simulink model "Uebung07_Aufgabe1_urspruengliche_Situation"  (R2017a)
settings: Solver=VariableStepAuto  StartTime=0.0  StopTime=10000  RelTol=1e-3  EnableMultiTasking=on
undefined symbols (not defined in the file or in its folder): calcElapsedTime, entity, m, n
settings Model: Creator=gome  LastModifiedBy=gome
settings OptimizationCC: LifeSpan=inf
settings DebuggingCC: SFUnexpectedBacktrackingDiag=warning  SFNoUnconditionalDefaultTransitionDiag=warning  SFExecutionAtInitializationDiag=none
settings GRTTargetCC: TargetLangStandard=C89/C90 (ANSI)  GeneratePreprocessorConditionals=Disable all
settings ConfigComp: CovMetricSettings=dw  CovHtmlReporting=on  CovSaveCumulativeToWorkspaceVar=on  CovSaveSingleToWorkspaceVar=on  CovExternalEMLEnable=off

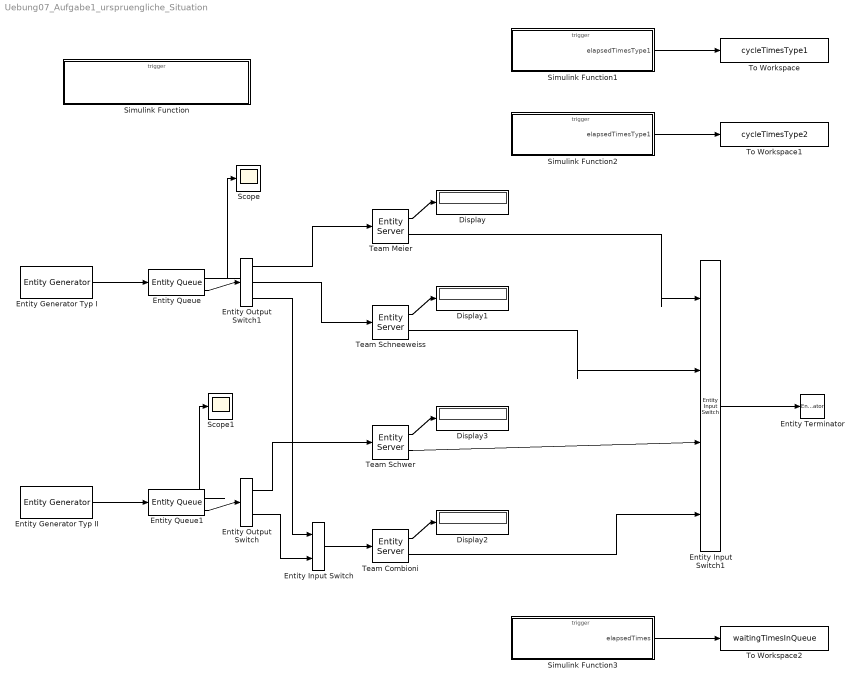
== system Uebung07_Aufgabe1_urspruengliche_Situation ==
  Display{,1..3} (4 alike) : Display
  Entity Input Switch : EntityInputSwitch  InputPortMessageModes=m,m  OutputPortMessageModes=m
  Entity Input Switch1 : EntityInputSwitch  InputPortMessageModes=m,m,m,m  OutputPortMessageModes=m  NumberInputPorts=4
      settings: InputPortMap=u1,u2,u3,u4
  Entity Output Switch : EntityOutputSwitch  InputPortMessageModes=m  OutputPortMessageModes=m,m  SwitchAttributeName=Attribute1
  Entity Output Switch1 : EntityOutputSwitch  InputPortMessageModes=m  OutputPortMessageModes=m,m,m  NumberOutputPorts=3  SwitchAttributeName=Attribute1
      settings: OutputPortMap=o0,o1,o2
  Entity Generator Typ I : EntityGenerator  OutputPortMessageModes=m  TimeSource=MATLAB action  IntergenerationTimeAction=dt = exprnd(0.333333);  GenerateAction=|  AttributeName=startTime|serviceTime|type  AttributeInitialValue=1|1|1  EntityType=Structured  EntityTypeName=Entity
      | entity.startTime = getCurrentSimTime;
      | entity.serviceTime = exprnd(0.25);
  Entity Generator Typ II : EntityGenerator  OutputPortMessageModes=m  TimeSource=MATLAB action  Period=36.3636  IntergenerationTimeAction=|  GenerateAction=|  AttributeName=startTime|serviceTime|type  AttributeInitialValue=1|1|2  EntityType=Structured  EntityTypeName=Entity
      IntergenerationTimeAction=|
      | persistent init
      | if isempty(init)
      |     init = 1;
      |     rng(845094850);
      | end
      | 
      | dt = exprnd(1.7143);
      GenerateAction=|
      | entity.startTime = getCurrentSimTime;
      | entity.serviceTime = exprnd(1);
  Entity Queue : EntityQueue  InputPortMessageModes=m  OutputPortMessageModes=n,m  Capacity=inf  ExitAction=calcElapsedTime(entity.startTime);  NumberEntitiesInBlock=on
      settings: OutputPortMap=o1,o5
  Entity Queue1 : EntityQueue  InputPortMessageModes=m  OutputPortMessageModes=n,m  Capacity=inf  ExitAction=calcElapsedTime(entity.startTime);  NumberEntitiesInBlock=on
      settings: OutputPortMap=o1,o5
  Entity Terminator : EntityTerminator  InputPortMessageModes=m  EntryAction=|
      | if entity.type == 1
      |     calcElapsedTime1(entity.startTime);
      | else
      |     calcElapsedTime2(entity.startTime);
      | end
  Scope : Scope
  Scope1 : Scope
  Simulink Function : Subsystem  TreatAsAtomicUnit=on
  Simulink Function1 : Subsystem  TreatAsAtomicUnit=on
  Simulink Function2 : Subsystem  TreatAsAtomicUnit=on
  Simulink Function3 : Subsystem  TreatAsAtomicUnit=on
  Team Combioni : EntityServer  InputPortMessageModes=m  OutputPortMessageModes=n,m  Capacity=1  ServiceTimeSource=Attribute  ServiceTimeAttributeName=serviceTime  Utilization=on
      settings: OutputPortMap=o5,o9
  Team Meier : EntityServer  InputPortMessageModes=m  OutputPortMessageModes=n,m  Capacity=1  ServiceTimeSource=Attribute  ServiceTimeAttributeName=serviceTime  Utilization=on
      settings: OutputPortMap=o5,o9
  Team Schneeweiss : EntityServer  InputPortMessageModes=m  OutputPortMessageModes=n,m  Capacity=1  ServiceTimeSource=Attribute  ServiceTimeAttributeName=serviceTime  Utilization=on
      settings: OutputPortMap=o5,o9
  Team Schwer : EntityServer  InputPortMessageModes=m  OutputPortMessageModes=n,m  Capacity=1  ServiceTimeSource=Attribute  ServiceTimeAttributeName=serviceTime  Utilization=on
      settings: OutputPortMap=o5,o9
  To Workspace : ToWorkspace  VariableName=cycleTimesType1  SaveFormat=Timeseries  SampleTime=-1
  To Workspace1 : ToWorkspace  VariableName=cycleTimesType2  SaveFormat=Timeseries  SampleTime=-1
  To Workspace2 : ToWorkspace  VariableName=waitingTimesInQueue  SaveFormat=Timeseries  SampleTime=-1
  wires:
  Entity Queue/2 -> Entity Output Switch1/1
  Entity Queue1/2 -> Entity Output Switch/1
  Entity Generator Typ II/1 -> Entity Queue1/1
  Entity Generator Typ I/1 -> Entity Queue/1
  Entity Output Switch1/1 -> Team Meier/1
  Entity Output Switch1/2 -> Team Schneeweiss/1
  Entity Input Switch/1 -> Team Combioni/1
  Entity Output Switch1/3 -> Entity Input Switch/1
  Entity Output Switch/2 -> Entity Input Switch/2
  Entity Output Switch/1 -> Team Schwer/1
  Team Meier/2 -> Entity Input Switch1/1
  Team Schneeweiss/2 -> Entity Input Switch1/2
  Team Schwer/2 -> Entity Input Switch1/3
  Team Combioni/2 -> Entity Input Switch1/4
  Entity Input Switch1/1 -> Entity Terminator/1
  Simulink Function1/1(elapsedTimesType1) -> To Workspace/1
  Team Meier/1 -> Display/1
  Team Combioni/1 -> Display2/1
  Team Schwer/1 -> Display3/1
  Team Schneeweiss/1 -> Display1/1
  Simulink Function2/1(elapsedTimesType1) -> To Workspace1/1
  Simulink Function3/1(elapsedTimes) -> To Workspace2/1
  Entity Queue/1 -> Scope/1
  Entity Queue1/1 -> Scope1/1

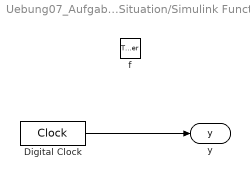
== system Uebung07_Aufgabe1_urspruengliche_Situation/Simulink Function ==
  f : TriggerPort  TriggerType=function-call  IsSimulinkFunction=on  FunctionName=getCurrentSimTime  VariantControl=Variant
  Digital Clock : DigitalClock  SampleTime=-1
  y : ArgOut  DisableCoverage=on  ArgumentName=y
  wires:
  Digital Clock/1 -> y/1

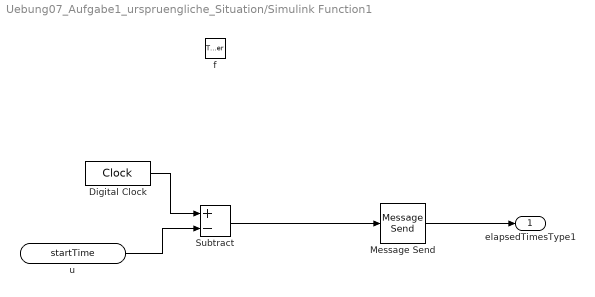
== system Uebung07_Aufgabe1_urspruengliche_Situation/Simulink Function1 ==
  f : TriggerPort  TriggerType=function-call  IsSimulinkFunction=on  FunctionName=calcElapsedTime1  VariantControl=Variant
  Digital Clock : DigitalClock  SampleTime=-1
  Message Send : MessageSend  OutputPortMessageModes=m
      settings: InputPortMap=u1
  Subtract : Sum  Inputs=+-
  u : ArgIn  DisableCoverage=on  ArgumentName=startTime
  elapsedTimesType1 : Outport
  wires:
  Message Send/1 -> elapsedTimesType1/1
  Subtract/1 -> Message Send/1
  Digital Clock/1 -> Subtract/1
  u/1 -> Subtract/2

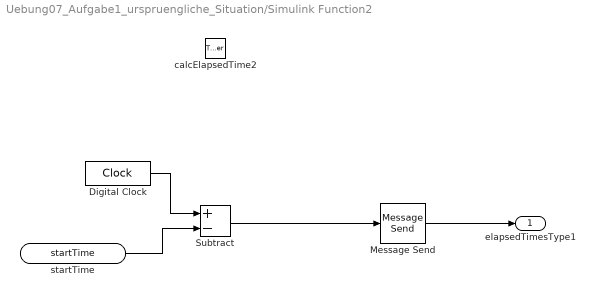
== system Uebung07_Aufgabe1_urspruengliche_Situation/Simulink Function2 ==
  calcElapsedTime2 : TriggerPort  TriggerType=function-call  IsSimulinkFunction=on  FunctionName=calcElapsedTime2  VariantControl=Variant
  Digital Clock : DigitalClock  SampleTime=-1
  Message Send : MessageSend  OutputPortMessageModes=m
      settings: InputPortMap=u1
  Subtract : Sum  Inputs=+-
  startTime : ArgIn  DisableCoverage=on  ArgumentName=startTime
  elapsedTimesType1 : Outport
  wires:
  Message Send/1 -> elapsedTimesType1/1
  Subtract/1 -> Message Send/1
  Digital Clock/1 -> Subtract/1
  startTime/1 -> Subtract/2

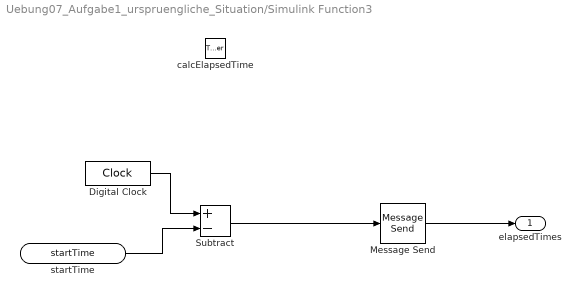
== system Uebung07_Aufgabe1_urspruengliche_Situation/Simulink Function3 ==
  calcElapsedTime : TriggerPort  TriggerType=function-call  IsSimulinkFunction=on  FunctionName=calcElapsedTime  VariantControl=Variant
  Digital Clock : DigitalClock  SampleTime=-1
  Message Send : MessageSend  OutputPortMessageModes=m
      settings: InputPortMap=u1
  Subtract : Sum  Inputs=+-
  startTime : ArgIn  DisableCoverage=on  ArgumentName=startTime
  elapsedTimes : Outport
  wires:
  Message Send/1 -> elapsedTimes/1
  Subtract/1 -> Message Send/1
  Digital Clock/1 -> Subtract/1
  startTime/1 -> Subtract/2
